simulink model "Fullsim_MPC"  (R2025b)
settings: Solver=ode4  StartTime=0.0  StopTime=100  FixedStep=0.01  RelTol=1e-3
undefined symbols (not defined in the file): psi_op, theta_op, V_mp_op, V_my_op, w_psi_op, w_theta_op
libraries: realtime_pacer_lib x1
settings Model: Creator=bulve  LastModifiedBy=Torstein
settings DebuggingCC: SignalInfNanChecking=error

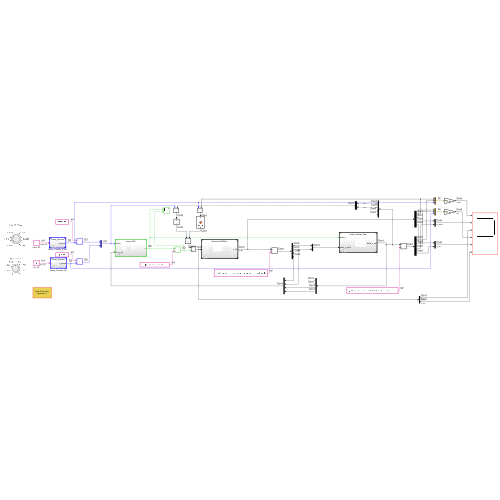
[thumbnail: Simulink's stored preview of the top-level diagram]
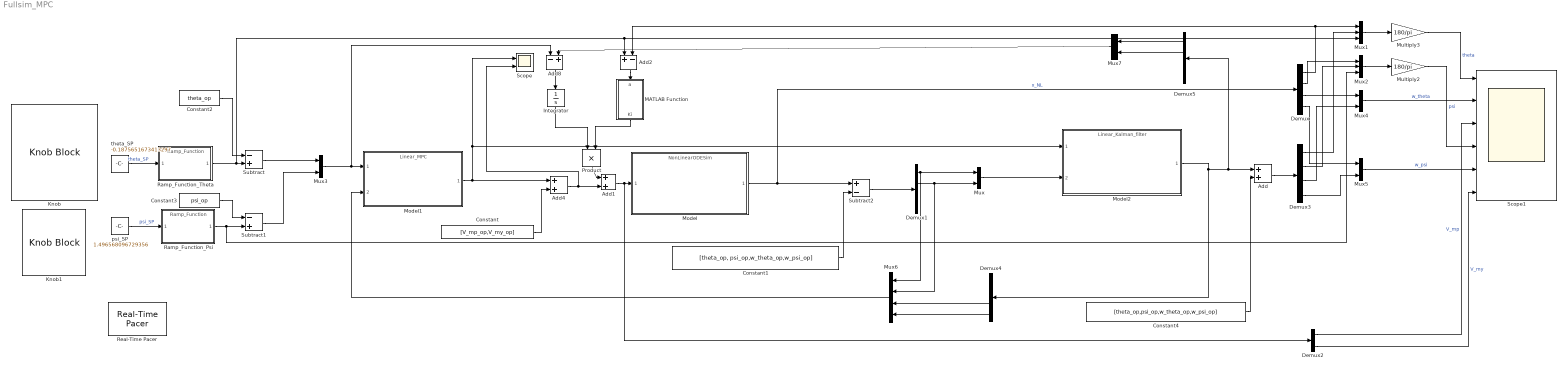
== system Fullsim_MPC ==
  Add : Sum
  Add1 : Sum
  Add2 : Sum  Inputs=+-
  Add4 : Sum
  Add8 : Sum  Inputs=-+
  Constant : Constant  Value=[V_mp_op,V_my_op]
  Constant1 : Constant  Value=[theta_op, psi_op,w_theta_op,w_psi_op]
  Constant2 : Constant  Value=theta_op
  Constant3 : Constant  Value=psi_op
  Constant4 : Constant  Value=[theta_op,psi_op,w_theta_op,w_psi_op]
  Demux{,1,3..5} (5 alike) : Demux
  Demux2 : Demux  Outputs=2
  Integrator : Integrator
  Knob : KnobBlock  ScaleMin=-0.6745  ScaleMax=0.3255
  Knob1 : KnobBlock  ScaleMin=1  ScaleMax=2
  MATLAB Function : MATLAB Function  TreatAsAtomicUnit=on
  Model : ModelReference  ModelNameDialog=NonLinearODESim.slx  SimulationMode=Normal  ModelReferenceVersion=2.1
  Model1 : ModelReference  ModelNameDialog=Linear_MPC.slx  SimulationMode=Normal  ModelReferenceVersion=1.33
  Model2 : ModelReference  ModelNameDialog=Linear_Kalman_filter.slx  SimulationMode=Normal  ModelReferenceVersion=1.20
  Multiply2 : Gain  Gain=180/pi
  Multiply3 : Gain  Gain=180/pi
  Mux{,3..5,7} (5 alike) : Mux  Inputs=2
  Mux1 : Mux  Inputs=3
  Mux2 : Mux  Inputs=3
  Mux6 : Mux
  Product : Product
  Ramp_Function_Psi : ModelReference  ModelNameDialog=Ramp_Function.slx  SimulationMode=Normal  ModelReferenceVersion=1.11
  Ramp_Function_Theta : ModelReference  ModelNameDialog=Ramp_Function.slx  SimulationMode=Normal  ModelReferenceVersion=1.11
  Real-Time Pacer : realtime_pacer_lib/Real-Time Pacer  simTimePerRealTime=1
      settings: SourceProductName=Real-Time Pacer
  Scope : Scope  NumInputPorts=2
      settings: ActiveDisplayYMinimum=-0.68755042727605353  ActiveDisplayYMaximum=1.2138082320511503
  Scope1 : Scope  NumInputPorts=6
      settings: ActiveDisplayYMinimum=-22.845823903284067  ActiveDisplayYMaximum=0.37993335089233904
  Subtract : Sum  Inputs=-+
  Subtract1 : Sum  Inputs=-+
  Subtract2 : Sum  Inputs=+-
  psi_SP : Constant  Value=1.496568096729356
  theta_SP : Constant  Value=-0.1875651673413297
  wires:
  psi_SP/1 -> Ramp_Function_Psi/1  "psi_SP"
  theta_SP/1 -> Ramp_Function_Theta/1  "theta_SP"
  Constant3/1 -> Subtract1/1
  Constant2/1 -> Subtract/1
  Mux3/1 -> Add8/1, Model1/1
  Add4/1 -> Add1/2, Scope/2
  Constant1/1 -> Subtract2/2
  Model2/1 -> Demux4/1, Demux5/1, Add/1
  Model1/1 -> Add4/1, Model2/1, Scope/1
  Constant/1 -> Add4/2
  Model/1 -> Subtract2/1, Demux/1  "x_NL"
  Mux2/1 -> Multiply2/1
  Mux1/1 -> Multiply3/1
  Demux/3 -> Mux4/1
  Constant4/1 -> Add/2
  Add/1 -> Demux3/1
  Demux3/3 -> Mux4/2
  Demux/4 -> Mux5/1
  Demux3/4 -> Mux5/2
  Multiply3/1 -> Scope1/1  "theta"
  Subtract/1 -> Mux3/1
  Subtract1/1 -> Mux3/2
  Subtract2/1 -> Demux1/1
  Demux1/1 -> Mux6/1, Mux/1
  Demux1/2 -> Mux6/2, Mux/2
  Mux/1 -> Model2/2
  Demux4/3 -> Mux6/3
  Demux4/4 -> Mux6/4
  Mux6/1 -> Model1/2
  Demux/1 -> Mux1/1, Add2/2
  Demux/2 -> Mux2/1
  Demux3/2 -> Mux2/2
  Demux3/1 -> Mux1/2
  Ramp_Function_Theta/1 -> Mux1/3, Add2/1, Subtract/2
  Ramp_Function_Psi/1 -> Mux2/3, Subtract1/2
  Demux2/1 -> Scope1/3  "V_mp"
  Multiply2/1 -> Scope1/4  "psi"
  Mux4/1 -> Scope1/2  "w_theta"
  Mux5/1 -> Scope1/5  "w_psi"
  Demux2/2 -> Scope1/6  "V_my"
  Add8/1 -> Integrator/1
  Integrator/1 -> Product/1
  Demux5/1 -> Mux7/1
  Demux5/2 -> Mux7/2
  Mux7/1 -> Add8/2
  Add1/1 -> Model/1, Demux2/1
  Product/1 -> Add1/1
  Add2/1 -> MATLAB Function/1(a)
  MATLAB Function/1(Ki) -> Product/2

== matlab function Fullsim_MPC/MATLAB Function ==
  data: a input; Ki output
function Ki = get_Ki(a)

Ki = -max(0.15, min(0.8, 3 * max(abs(a))));
